simulink model "UAVLinCL_tracking_Hramp"  (R2023a)
settings: Solver=VariableStepAuto  StartTime=0.0  StopTime=40  RelTol=1e-3
values from neighbouring files (symbols this model uses):
  A = [-0.5572,-0.7814;0.7814,0]    [Calculos02_Vnoladetrim.m]
  B = [1,-1;0,2]    [Calculos02_Vnoladetrim.m]
  C = [1.9691,6.4493]    [Calculos02_Vnoladetrim.m]
  Ct = [0, 0, 0, 0, 1]    [PI_6_Tracker_GS.m]    (also in PI_6_Tracker_bigGuy.m)
  K1 = Kt(:,1:5)    [PI_6_Tracker_GS.m]    (also in PI_6_Tracker_bigGuy.m)
  K2 = Kt(:,6)    [PI_6_Tracker_GS.m]    (also in PI_6_Tracker_bigGuy.m)
  rampH = Vstart*tan(path_angle*pi/180)    [PI_6_Tracker_GS.m]    (also in PI_6_Tracker_bigGuy.m = Vs_trim_range*tan(path_angle*pi/180))
  x0t = zeros(5,1)    [PI_6_Tracker_GS.m]    (also in PI_6_Tracker_bigGuy.m)
undefined symbols (not defined in the file or in its folder): D, Utrim
libraries: simulink x2
settings Model: Creator=Nacho  LastModifiedBy=ignac
settings SolverCC: AlgebraicLoopSolver=TrustRegion
settings DebuggingCC: UnconnectedInputMsg=warning  UnconnectedOutputMsg=warning  UnconnectedLineMsg=warning
settings ModelReferenceCC: EnableRefExpFcnMdlSchedulingChecks=on
settings RTWCC: DLArmComputeVersion=19.05

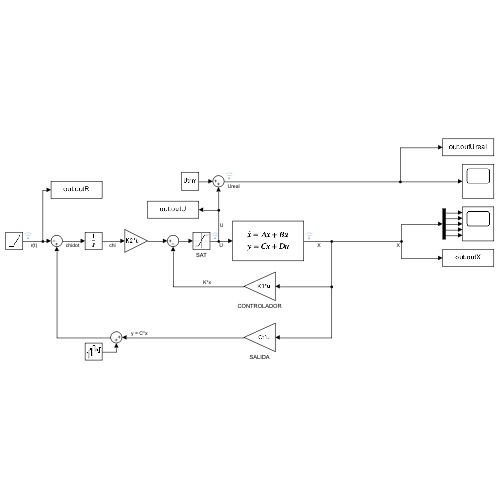
[thumbnail: Simulink's stored preview of the top-level diagram]
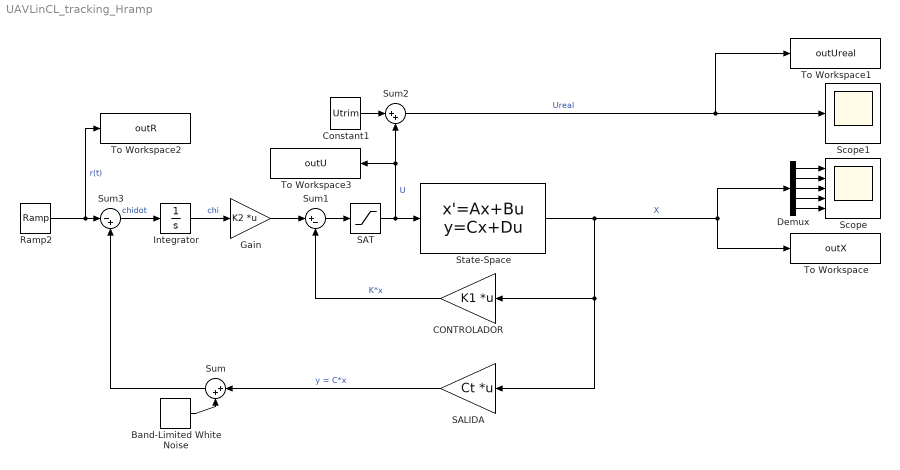
== system UAVLinCL_tracking_Hramp ==
  Band-Limited White Noise : simulink/Sources/Band-Limited White Noise  Cov=[0.1]*0  Ts=0.1  seed=[23341]
  CONTROLADOR : Gain  Gain=K1  Multiplication=Matrix(K*u)
  Constant1 : Constant  Value=Utrim
  Demux : Demux  Outputs=5
  Gain : Gain  Gain=K2  Multiplication=Matrix(K*u)
  Integrator : Integrator
  Ramp2 : simulink/Sources/Ramp  slope=rampH  start=0  InitialOutput=0
  SALIDA : Gain  Gain=Ct  Multiplication=Matrix(K*u)
  SAT : Saturate  UpperLimit=[1; 0.5] - Utrim  LowerLimit=[0; -0.5] - Utrim
  Scope : Scope  NumInputPorts=5
  Scope1 : Scope
  State-Space : StateSpace  A=A  B=B  C=C  D=D  InitialCondition=x0t
  Sum : Sum  Inputs=|++
  Sum1 : Sum  Inputs=|+-
  Sum2 : Sum  Inputs=|++
  Sum3 : Sum  Inputs=|-+
  To Workspace : ToWorkspace  VariableName=outX  SampleTime=-1
      settings: Save2DSignal=2-D array (concatenate along first dimension)
  To Workspace1 : ToWorkspace  VariableName=outUreal  SampleTime=-1
      settings: Save2DSignal=2-D array (concatenate along first dimension)
  To Workspace2 : ToWorkspace  VariableName=outR  SampleTime=-1
      settings: Save2DSignal=2-D array (concatenate along first dimension)
  To Workspace3 : ToWorkspace  VariableName=outU  SampleTime=-1
  wires:
  Demux/1 -> Scope/1
  Demux/2 -> Scope/2
  Demux/4 -> Scope/4
  Demux/3 -> Scope/3
  State-Space/1 -> To Workspace/1, Demux/1, CONTROLADOR/1, SALIDA/1  "X"
  CONTROLADOR/1 -> Sum1/2  "K*x"
  Constant1/1 -> Sum2/1
  Sum2/1 -> To Workspace1/1, Scope1/1  "Ureal"
  Ramp2/1 -> To Workspace2/1, Sum3/1  "r(t)"
  SALIDA/1 -> Sum/1  "y = C*x"
  Sum3/1 -> Integrator/1  "chidot"
  Integrator/1 -> Gain/1  "chi"
  Gain/1 -> Sum1/1
  Sum1/1 -> SAT/1
  SAT/1 -> To Workspace3/1, Sum2/2, State-Space/1  "U"
  Demux/5 -> Scope/5
  Band-Limited White Noise/1 -> Sum/2
  Sum/1 -> Sum3/2
